simulink model "MIL_VehicleTestEnvironment_MG_DCT_19a"  (Simulink 9.3)
settings: Solver=ode4  StartTime=0.0  StopTime=20  FixedStep=0.001  MaxStep=0.005  RelTol=1e-3  EnableMultiTasking=on
model workspace (MAT data in the model file):
  CGFrntAxleDist = Simulink.Parameter
  CGFrntAxleDist.Value = 1.024
  CGFrntAxleDist.Description = ' the longitudinal distance from the center of gravity to front axle, [m]'
  CGFrntAxleDist.DataType = 'auto'
  CGFrntAxleDist.Dimensions = [1 1]
  CGHght = Simulink.Parameter
  CGHght.Value = 0.654
  CGHght.Description = 'the height of the center of gravity from ground, [m]'
  CGHght.DataType = 'auto'
  CGHght.Dimensions = [1 1]
  CGRearAxleDist = Simulink.Parameter
  CGRearAxleDist.Value = 1.536
  CGRearAxleDist.Description = 'the longitudinal distance from the center of gravity to rear axle, [m]'
  CGRearAxleDist.DataType = 'auto'
  CGRearAxleDist.Dimensions = [1 1]
  Clu1EffRad = Simulink.Parameter
  Clu1EffRad.Value = 0.1847
  Clu1EffRad.Description = 'the diameter of outer circle of clutch 1, [m]'
  Clu1EffRad.DataType = 'auto'
  Clu1EffRad.Dimensions = [1 1]
  Clu1FricCoefMap = Simulink.Parameter
  Clu1FricCoefMap.Value = [0  0.11; 100  0.1221; 300  0.1266; 1000  0.1348; 1700  0.1435]
  Clu1FricCoefMap.Description = 'the friction coefficent of clutch 1 as a function of angular velocity difference [rpm]'
  Clu1FricCoefMap.DataType = 'auto'
  Clu1FricCoefMap.Dimensions = [5 2]
  Clu1FricSurfNum = Simulink.Parameter
  Clu1FricSurfNum.Value = 6
  Clu1FricSurfNum.Description = 'the amount of friction surfaces on clutch 1'
  Clu1FricSurfNum.DataType = 'auto'
  Clu1FricSurfNum.Dimensions = [1 1]
  Clu1OutpInrt = Simulink.Parameter
  Clu1OutpInrt.Value = 0.003321
  Clu1OutpInrt.Description = 'inertia of Clutch output part 1, [kg*m*m]'
  Clu1OutpInrt.DataType = 'auto'
  Clu1OutpInrt.Dimensions = [1 1]
  Clu1PMin = Simulink.Parameter
  Clu1PMin.Value = 1.3
  Clu1PMin.DataType = 'auto'
  Clu1PMin.Dimensions = [1 1]
  Clu1PresArea = Simulink.Parameter
  Clu1PresArea.Value = 0.0035
  Clu1PresArea.Description = 'the effected area of the oil pressure on clutch 1, [m*m] '
  Clu1PresArea.DataType = 'auto'
  Clu1PresArea.Dimensions = [1 1]
  Clu1SprFor = Simulink.Parameter
  Clu1SprFor.Value = 809
  Clu1SprFor.Description = 'the seperate spring force of clutch 1, [N]'
  Clu1SprFor.DataType = 'auto'
  Clu1SprFor.Dimensions = [1 1]
  Clu1StatFricCoef = Simulink.Parameter
  Clu1StatFricCoef.Value = 0.12
  Clu1StatFricCoef.Description = 'the static friction peak coefficient of clutch 2, no less than the kinetic friction coefficient at 0 velocity'
  Clu1StatFricCoef.DataType = 'auto'
  Clu1StatFricCoef.Dimensions = [1 1]
  Clu2EffRad = Simulink.Parameter
  Clu2EffRad.Value = 0.1397
  Clu2EffRad.Description = 'the effected radius of clutch 2, [m]'
  Clu2EffRad.DataType = 'auto'
  Clu2EffRad.Dimensions = [1 1]
  Clu2FricCoefMap = Simulink.Parameter
  Clu2FricCoefMap.Value = [0  0.11; 100  0.1225; 300  0.1274; 1000  0.1348; 1700  0.1397]
  Clu2FricCoefMap.Description = 'the friction coefficent of clutch 2 as a function of angular velocity difference [rpm]'
  Clu2FricCoefMap.DataType = 'auto'
  Clu2FricCoefMap.Dimensions = [5 2]
  Clu2FricSurfNum = Simulink.Parameter
  Clu2FricSurfNum.Value = 8
  Clu2FricSurfNum.Description = 'the amount of friction surfaces on clutch 2'
  Clu2FricSurfNum.DataType = 'auto'
  Clu2FricSurfNum.Dimensions = [1 1]
  Clu2OutpInrt = Simulink.Parameter
  Clu2OutpInrt.Value = 0.002617
  Clu2OutpInrt.Description = 'inertia of Clutch output part 2, [kg*m*m]'
  Clu2OutpInrt.DataType = 'auto'
  Clu2OutpInrt.Dimensions = [1 1]
  Clu2PMin = Simulink.Parameter
  Clu2PMin.Value = 1.3
  Clu2PMin.DataType = 'auto'
  Clu2PMin.Dimensions = [1 1]
  Clu2PresArea = Simulink.Parameter
  Clu2PresArea.Value = 0.0035
  Clu2PresArea.Description = 'the effected area of the oil pressure on clutch 2, [m*m] '
  Clu2PresArea.DataType = 'auto'
  Clu2PresArea.Dimensions = [1 1]
  Clu2SprFor = Simulink.Parameter
  Clu2SprFor.Value = 809
  Clu2SprFor.Description = 'the seperate spring force of clutch 2, [N]'
  Clu2SprFor.DataType = 'auto'
  Clu2SprFor.Dimensions = [1 1]
  Clu2StatFricCoef = Simulink.Parameter
  Clu2StatFricCoef.Value = 0.12
  Clu2StatFricCoef.Description = 'the static friction peak coefficient of clutch 2, no less than the kinetic friction coefficient at 0 velocity'
  Clu2StatFricCoef.DataType = 'auto'
  Clu2StatFricCoef.Dimensions = [1 1]
  CluInpInrt = Simulink.Parameter
  CluInpInrt.Value = 0.0225
  CluInpInrt.Description = 'inertia of Clutch input part, [kg*m*m]'
  CluInpInrt.DataType = 'auto'
  CluInpInrt.Dimensions = [1 1]
  CluSoln1LineI = Simulink.Parameter
  CluSoln1LineI.Value = [200 400 600 800 950]
  CluSoln1LineI.Description = 'mA
    | '
  CluSoln1LineI.DataType = 'auto'
  CluSoln1LineI.Dimensions = [1 5]
  CluSoln1LineP = Simulink.Parameter
  CluSoln1LineP.Value = [0 2.5 8.85 15.77 20]
  CluSoln1LineP.Description = 'bar/1000'
  CluSoln1LineP.DataType = 'auto'
  CluSoln1LineP.Dimensions = [1 5]
  CluSoln2LineI = Simulink.Parameter
  CluSoln2LineI.Value = [200 400 600 800 950]
  CluSoln2LineI.Description = 'mA
    | '
  CluSoln2LineI.DataType = 'auto'
  CluSoln2LineI.Dimensions = [1 5]
  CluSoln2LineP = Simulink.Parameter
  CluSoln2LineP.Value = [0 2.5 8.85 15.77 20]
  CluSoln2LineP.Description = 'bar/1000'
  CluSoln2LineP.DataType = 'auto'
  CluSoln2LineP.Dimensions = [1 5]
  DiffDampCoef = Simulink.Parameter
  DiffDampCoef.Value = 0.001
  DiffDampCoef.Description = 'the inertia of final drive gear and differential, [kg*m*m]'
  DiffDampCoef.DataType = 'auto'
  DiffDampCoef.Dimensions = [1 1]
  DiffInrt = Simulink.Parameter
  DiffInrt.Value = 0.0448
  DiffInrt.Description = 'the inertia of final drive gear and differential, [kg*m*m]'
  DiffInrt.DataType = 'auto'
  DiffInrt.Dimensions = [1 1]
  EngDampCoef = Simulink.Parameter
  EngDampCoef.Value = 0.03
  EngDampCoef.Description = 'the damper coefficent of engine shaft, [N*m*s/rad]'
  EngDampCoef.DataType = 'auto'
  EngDampCoef.Dimensions = [1 1]
  EngFuelCnsPerKWhMapCns = Simulink.Parameter
  EngFuelCnsPerKWhMapCns.Value = [300 300 300 300 300 300 300 300 300 300 300 300 ... (5858 elements, 101x58)]
  EngFuelCnsPerKWhMapCns.DataType = 'auto'
  EngFuelCnsPerKWhMapCns.Dimensions = [101 58]
  EngFuelCnsPerKWhMapSpdIndx = Simulink.Parameter
  EngFuelCnsPerKWhMapSpdIndx.Value = [800 900 1000 1100 1200 1300 1400 1500 1600 1700 1800 1900 2000 2100 2200 2300 2400 2500 2600 2700 2800 2900 3000 3100 3200 3300 3400 3500 3600 3700 3800 3900 4000 4100 4200 4300 4400 4500 4600 4700 4800 4900 5000 5100 5200 5300 5400 5500 5600 5700 5800 5900 6000 6100 6200 6300 6400 6500]
  EngFuelCnsPerKWhMapSpdIndx.DataType = 'auto'
  EngFuelCnsPerKWhMapSpdIndx.Dimensions = [1 58]
  EngFuelCnsPerKWhMapThrtIndx = Simulink.Parameter
  EngFuelCnsPerKWhMapThrtIndx.Value = [0 1 2 3 4 5 6 7 8 9 10 11 12 13 14 15 16 17 18 19 20 21 22 23 24 25 26 27 28 29 30 31 32 33 34 35 36 37 38 39 40 41 42 43 44 45 46 47 48 49 50 51 52 53 54 55 56 57 58 59 60 61 62 63 64 65 66 67 68 69 70 71 72 73 74 75 76 77 78 79 80 81 82 83 84 85 86 87 88 89 90 91 92 93 94 95 96 97 98 99 100]
  EngFuelCnsPerKWhMapThrtIndx.DataType = 'auto'
  EngFuelCnsPerKWhMapThrtIndx.Dimensions = [1 101]
  EngFuelCnsPerSecMapCns = Simulink.Parameter
  EngFuelCnsPerSecMapCns.Value = [0.08 0.2 0.3 0.32 0.34 0.37 0.39 0.41 0.43 0.46 0.48 0.5 ... (494 elements, 26x19)]
  EngFuelCnsPerSecMapCns.DataType = 'auto'
  EngFuelCnsPerSecMapCns.Dimensions = [26 19]
  EngFuelCnsPerSecMapSpdIndx = Simulink.Parameter
  EngFuelCnsPerSecMapSpdIndx.Value = [600 800 1000 1200 1400 1600 1800 2000 2200 2400 2800 3200 3600 4000 4400 4800 5200 5600 5800]
  EngFuelCnsPerSecMapSpdIndx.DataType = 'auto'
  EngFuelCnsPerSecMapSpdIndx.Dimensions = [1 19]
  EngFuelCnsPerSecMapThrtIndx = Simulink.Parameter
  EngFuelCnsPerSecMapThrtIndx.Value = [0 4 8 12 16 20 24 28 32 36 40 44 48 52 56 60 64 68 72 76 80 84 88 92 96 100]
  EngFuelCnsPerSecMapThrtIndx.DataType = 'auto'
  EngFuelCnsPerSecMapThrtIndx.Dimensions = [1 26]
  EngFuelRateMapPwrIndx = Simulink.Parameter
  EngFuelRateMapPwrIndx.Value = [0 1 2 3 4 5 6 7 8 9 10 11 12 13 14 15 16 17 18 19 20 21 22 23 24 25 26 27 28 29 30 31 32 33 34 35 36 37 38 39 40 41 42 43 44 45 46 47 48 49 50 51 52 53 54 55 56 57 58 59 60 61 62 63 64 65 66 67 68 69 70 71 72 73 74 75 76 77 78 79 80 81 82 83 84 85 86 87 88 89 90 91 92 93 94 95 96 97 98 99 100 101 102 103 104 105 106 107 108 109 110 111 112 113 114 115 116 117 118 119 120 121 122 123 124 125 126 127 128 129 130 131 132 133 134 135 136 137 138 139 140 141 142 143 144 145 146 147 148 149 150 151 152 153 154 155 156 157 158 159 160 161]
  EngFuelRateMapPwrIndx.DataType = 'auto'
  EngFuelRateMapPwrIndx.Dimensions = [1 162]
  EngFuelRateMapRate = Simulink.Parameter
  EngFuelRateMapRate.Value = [299.999982085 300.000046004 299.999957683 299.999715746 300.001791195 299.994024584 300.011592336 299.999851192 299.918999195 299.430328902 286.286371749 262.121506938 ... (9396 elements, 162x58)]
  EngFuelRateMapRate.DataType = 'auto'
  EngFuelRateMapRate.Dimensions = [162 58]
  EngFuelRateMapSpdIndx = Simulink.Parameter
  EngFuelRateMapSpdIndx.Value = [800 900 1000 1100 1200 1300 1400 1500 1600 1700 1800 1900 2000 2100 2200 2300 2400 2500 2600 2700 2800 2900 3000 3100 3200 3300 3400 3500 3600 3700 3800 3900 4000 4100 4200 4300 4400 4500 4600 4700 4800 4900 5000 5100 5200 5300 5400 5500 5600 5700 5800 5900 6000 6100 6200 6300 6400 6500]
  EngFuelRateMapSpdIndx.DataType = 'auto'
  EngFuelRateMapSpdIndx.Dimensions = [1 58]
  EngIdleSpd = Simulink.Parameter
  EngIdleSpd.Value = 750
  EngIdleSpd.Description = 'the rated idle speed of engine, [rpm]'
  EngIdleSpd.DataType = 'auto'
  EngIdleSpd.Dimensions = [1 1]
  EngInrt = Simulink.Parameter
  EngInrt.Value = 0.2
  EngInrt.Description = 'the inertia of engine crank shaft and flywheel, [kg*m*m] '
  EngInrt.DataType = 'auto'
  EngInrt.Dimensions = [1 1]
  EngPwrMax = Simulink.Parameter
  EngPwrMax.Value = 162
  EngPwrMax.Description = ' maximum engine power, [kW]'
  EngPwrMax.DataType = 'auto'
  EngPwrMax.Dimensions = [1 1]
  EngSpdMax = Simulink.Parameter
  EngSpdMax.Value = 6500
  EngSpdMax.Description = 'maximum engine speed, [rpm]'
  EngSpdMax.DataType = 'auto'
  EngSpdMax.Dimensions = [1 1]
  EngTqExtChartc = Simulink.Parameter
  EngTqExtChartc.Value = [0 0 118.17 213.22 253 289.28 303.52 321 337.08 350 350 350 350 350 337.32 323.08 306.7 267.43 228.27 144 -80]
  EngTqExtChartc.DataType = 'auto'
  EngTqExtChartc.Dimensions = [1 21]
  EngTqMapSpdIndx = Simulink.Parameter
  EngTqMapSpdIndx.Value = [0 400 517 633 750 1107 1463 1820 2177 2533 2890 3247 3603 3960 4317 4673 5030 5387 5743 6100 6500]
  EngTqMapSpdIndx.Description = 'the speed index of engine universal characteristics, [rpm]'
  EngTqMapSpdIndx.DataType = 'auto'
  EngTqMapSpdIndx.Dimensions = [1 21]
  EngTqMapThrtIndx = Simulink.Parameter
  EngTqMapThrtIndx.Value = [0 10 20 30 40 50 60 70 80 90 100]
  EngTqMapThrtIndx.Description = 'the throttle index of engine universal characteristics, [%]'
  EngTqMapThrtIndx.DataType = 'auto'
  EngTqMapThrtIndx.Dimensions = [1 11]
  EngTqMapTq = Simulink.Parameter
  EngTqMapTq.Value = [0 0 0 0 0 0 0 0 0 0 0 0 ... (231 elements, 11x21)]
  EngTqMapTq.Description = 'torque map of engine universal characteristics, 11*20, [Nm]'
  EngTqMapTq.DataType = 'auto'
  EngTqMapTq.Dimensions = [11 21]
  EngTqMax = Simulink.Parameter
  EngTqMax.Value = 350
  EngTqMax.Description = 'maximum torque of engine, [Nm]'
  EngTqMax.DataType = 'auto'
  EngTqMax.Dimensions = [1 1]
  FinlGearRat1 = Simulink.Parameter
  FinlGearRat1.Value = 4.28
  FinlGearRat1.Description = 'the gear ratio of final drive 1'
  FinlGearRat1.DataType = 'auto'
  FinlGearRat1.Dimensions = [1 1]
  FinlGearRat2 = Simulink.Parameter
  FinlGearRat2.Value = 2.85
  FinlGearRat2.Description = 'the gear ratio of final drive 2'
  FinlGearRat2.DataType = 'auto'
  FinlGearRat2.Dimensions = [1 1]
  Fork13ActrAr = Simulink.Parameter
  Fork13ActrAr.Value = 400
  Fork13ActrAr.Description = 'mm^2'
  Fork13ActrAr.DataType = 'auto'
  Fork13ActrAr.Dimensions = [1 1]
  Fork1PosnA = Simulink.Parameter
  Fork1PosnA.Value = 795
  Fork1PosnA.DataType = 'uint16'
  Fork1PosnA.Dimensions = [1 1]
  Fork1PosnB = Simulink.Parameter
  Fork1PosnB.Value = 249
  Fork1PosnB.DataType = 'uint16'
  Fork1PosnB.Dimensions = [1 1]
  Fork1PosnNeut = Simulink.Parameter
  Fork1PosnNeut.Value = 513
  Fork1PosnNeut.DataType = 'uint16'
  Fork1PosnNeut.Dimensions = [1 1]
  Fork1PosnSyncA = Simulink.Parameter
  Fork1PosnSyncA.Value = 630
  Fork1PosnSyncA.DataType = 'uint16'
  Fork1PosnSyncA.Dimensions = [1 1]
  Fork1PosnSyncB = Simulink.Parameter
  Fork1PosnSyncB.Value = 410
  Fork1PosnSyncB.DataType = 'uint16'
  Fork1PosnSyncB.Dimensions = [1 1]
  Fork24ActrAr = Simulink.Parameter
  Fork24ActrAr.Value = 400
  Fork24ActrAr.DataType = 'auto'
  Fork24ActrAr.Dimensions = [1 1]
  Fork2PosnA = Simulink.Parameter
  Fork2PosnA.Value = 798
  Fork2PosnA.DataType = 'uint16'
  Fork2PosnA.Dimensions = [1 1]
  Fork2PosnB = Simulink.Parameter
  Fork2PosnB.Value = 228
  Fork2PosnB.DataType = 'uint16'
  Fork2PosnB.Dimensions = [1 1]
  Fork2PosnNeut = Simulink.Parameter
  Fork2PosnNeut.Value = 495
  Fork2PosnNeut.DataType = 'uint16'
  Fork2PosnNeut.Dimensions = [1 1]
  Fork2PosnSyncA = Simulink.Parameter
  Fork2PosnSyncA.Value = 610
  Fork2PosnSyncA.DataType = 'uint16'
  Fork2PosnSyncA.Dimensions = [1 1]
  Fork2PosnSyncB = Simulink.Parameter
  Fork2PosnSyncB.Value = 390
  Fork2PosnSyncB.DataType = 'uint16'
  Fork2PosnSyncB.Dimensions = [1 1]
  Fork3PosnA = Simulink.Parameter
  Fork3PosnA.Value = 820
  Fork3PosnA.DataType = 'uint16'
  Fork3PosnA.Dimensions = [1 1]
  Fork3PosnB = Simulink.Parameter
  Fork3PosnB.Value = 218
  Fork3PosnB.DataType = 'uint16'
  Fork3PosnB.Dimensions = [1 1]
  Fork3PosnNeut = Simulink.Parameter
  Fork3PosnNeut.Value = 515
  Fork3PosnNeut.DataType = 'uint16'
  Fork3PosnNeut.Dimensions = [1 1]
  Fork3PosnSyncA = Simulink.Parameter
  Fork3PosnSyncA.Value = 630
  Fork3PosnSyncA.DataType = 'uint16'
  Fork3PosnSyncA.Dimensions = [1 1]
  Fork3PosnSyncB = Simulink.Parameter
  Fork3PosnSyncB.Value = 410
  Fork3PosnSyncB.DataType = 'uint16'
  Fork3PosnSyncB.Dimensions = [1 1]
  Fork4PosnA = Simulink.Parameter
  Fork4PosnA.Value = 810
  Fork4PosnA.DataType = 'uint16'
  Fork4PosnA.Dimensions = [1 1]
  Fork4PosnB = Simulink.Parameter
  Fork4PosnB.Value = 224
  Fork4PosnB.DataType = 'uint16'
  Fork4PosnB.Dimensions = [1 1]
  Fork4PosnNeut = Simulink.Parameter
  Fork4PosnNeut.Value = 513
  Fork4PosnNeut.DataType = 'uint16'
  Fork4PosnNeut.Dimensions = [1 1]
  Fork4PosnSyncA = Simulink.Parameter
  Fork4PosnSyncA.Value = 630
  Fork4PosnSyncA.DataType = 'uint16'
  Fork4PosnSyncA.Dimensions = [1 1]
  Fork4PosnSyncB = Simulink.Parameter
  Fork4PosnSyncB.Value = 410
  Fork4PosnSyncB.DataType = 'uint16'
  Fork4PosnSyncB.Dimensions = [1 1]
  Fork6RActrAr = Simulink.Parameter
  Fork6RActrAr.Value = 400
  Fork6RActrAr.Description = 'mm^2'
  Fork6RActrAr.DataType = 'auto'
  Fork6RActrAr.Dimensions = [1 1]
  ForkMass = Simulink.Parameter
  ForkMass.Value = 0.5
  ForkMass.Description = 'the mass of fork and fork shaft'
  ForkMass.DataType = 'auto'
  ForkMass.Dimensions = [1 1]
  ForkN5ActrAr = Simulink.Parameter
  ForkN5ActrAr.Value = 400
  ForkN5ActrAr.Description = 'mm^2'
  ForkN5ActrAr.DataType = 'auto'
  ForkN5ActrAr.Dimensions = [1 1]
  GearRat = Simulink.Parameter
  GearRat.Value = [3.25 1.88 1.21 0.9 1.03 0.79 4.33]
  GearRat.Description = 'the gear ratio at gear 1-7&R'
  GearRat.DataType = 'auto'
  GearRat.Dimensions = [1 7]
  HalfShafInrt = Simulink.Parameter
  HalfShafInrt.Value = 0.0068
  HalfShafInrt.Description = 'inertia of two half shaft, [kg*m*m]'
  HalfShafInrt.DataType = 'auto'
  HalfShafInrt.Dimensions = [1 1]
  IdleGearInrt = Simulink.Parameter
  IdleGearInrt.Value = [0.00367 0.00297 0.0018 0.00123 0.00086 0.00056 0.0018]
  IdleGearInrt.Description = '% inertia of idle gear of gear 1-7&R, [kg*m*m]'
  IdleGearInrt.DataType = 'auto'
  IdleGearInrt.Dimensions = [1 7]
  InpShaf1DampCoef = Simulink.Parameter
  InpShaf1DampCoef.Value = 0.001
  InpShaf1DampCoef.DataType = 'auto'
  InpShaf1DampCoef.Dimensions = [1 1]
  InpShaf1Inrt = Simulink.Parameter
  InpShaf1Inrt.Value = 0.0046
  InpShaf1Inrt.Description = 'the inertia of input shaft 1, including the gears on the shaft, [kg*m*m]'
  InpShaf1Inrt.DataType = 'auto'
  InpShaf1Inrt.Dimensions = [1 1]
  InpShaf2DampCoef = Simulink.Parameter
  InpShaf2DampCoef.Value = 0.001
  InpShaf2DampCoef.DataType = 'auto'
  InpShaf2DampCoef.Dimensions = [1 1]
  InpShaf2Inrt = Simulink.Parameter
  InpShaf2Inrt.Value = 0.0033
  InpShaf2Inrt.Description = ' the inertia of input shaft 2, including the gears on the shaft, [kg*m*m]'
  InpShaf2Inrt.DataType = 'auto'
  InpShaf2Inrt.Dimensions = [1 1]
  OutpShaf1DampCoef = Simulink.Parameter
  OutpShaf1DampCoef.Value = 0.001
  OutpShaf1DampCoef.DataType = 'auto'
  OutpShaf1DampCoef.Dimensions = [1 1]
  OutpShaf1Inrt = Simulink.Parameter
  OutpShaf1Inrt.Value = 0.0062
  OutpShaf1Inrt.Description = 'the inertia of output shaft 1, [kg*m*m]'
  OutpShaf1Inrt.DataType = 'auto'
  OutpShaf1Inrt.Dimensions = [1 1]
  OutpShaf2DampCoef = Simulink.Parameter
  OutpShaf2DampCoef.Value = 0.001
  OutpShaf2DampCoef.DataType = 'auto'
  OutpShaf2DampCoef.Dimensions = [1 1]
  OutpShaf2Inrt = Simulink.Parameter
  OutpShaf2Inrt.Value = 0.0085
  OutpShaf2Inrt.Description = 'the inertia of output shaft 2, [kg*m*m]'
  OutpShaf2Inrt.DataType = 'auto'
  OutpShaf2Inrt.Dimensions = [1 1]
  RoadSlop = Simulink.Parameter
  RoadSlop.Value = 0
  RoadSlop.Description = 'road slop gradient, [deg]'
  RoadSlop.DataType = 'auto'
  RoadSlop.Dimensions = [1 1]
  ShiftSoln1LineI = Simulink.Parameter
  ShiftSoln1LineI.Value = [0 1000 2000]
  ShiftSoln1LineI.Description = 'mA
    | '
  ShiftSoln1LineI.DataType = 'auto'
  ShiftSoln1LineI.Dimensions = [1 3]
  ShiftSoln1LineP = Simulink.Parameter
  ShiftSoln1LineP.Value = [0 10 20]
  ShiftSoln1LineP.Description = 'bar/1000'
  ShiftSoln1LineP.DataType = 'auto'
  ShiftSoln1LineP.Dimensions = [1 3]
  ShiftSoln2LineI = Simulink.Parameter
  ShiftSoln2LineI.Value = [0 1000 2000]
  ShiftSoln2LineI.Description = 'mA
    | '
  ShiftSoln2LineI.DataType = 'auto'
  ShiftSoln2LineI.Dimensions = [1 3]
  ShiftSoln2LineP = Simulink.Parameter
  ShiftSoln2LineP.Value = [0 10 20]
  ShiftSoln2LineP.Description = 'bar/1000'
  ShiftSoln2LineP.DataType = 'auto'
  ShiftSoln2LineP.Dimensions = [1 3]
  SynrConeAngl = Simulink.Parameter
  SynrConeAngl.Value = 5
  SynrConeAngl.Description = 'the cone angle of a synchronizer, [rad]
    | 7.5'
  SynrConeAngl.DataType = 'auto'
  SynrConeAngl.Dimensions = [1 1]
  SynrDetnForMax = Simulink.Parameter
  SynrDetnForMax.Value = 70
  SynrDetnForMax.Description = 'peak force of synchronizer''s detent, [N]'
  SynrDetnForMax.DataType = 'auto'
  SynrDetnForMax.Dimensions = [1 1]
  SynrDiaBig = Simulink.Parameter
  SynrDiaBig.Value = 0.0728
  SynrDiaBig.Description = 'the maximum diameter of synchronizer contact surface, [m]'
  SynrDiaBig.DataType = 'auto'
  SynrDiaBig.Dimensions = [1 1]
  SynrDiaSmal = Simulink.Parameter
  SynrDiaSmal.Value = 0.0676
  SynrDiaSmal.Description = 'the minimum diameter of synchronizer contact surface, [m]'
  SynrDiaSmal.DataType = 'auto'
  SynrDiaSmal.Dimensions = [1 1]
  SynrDplDog = Simulink.Parameter
  SynrDplDog.Value = 10.514
  SynrDplDog.DataType = 'auto'
  SynrDplDog.Dimensions = [1 1]
  SynrDplEngd = Simulink.Parameter
  SynrDplEngd.Value = 13.514
  SynrDplEngd.DataType = 'auto'
  SynrDplEngd.Dimensions = [1 1]
  SynrDplFinshd = Simulink.Parameter
  SynrDplFinshd.Value = 18.211
  SynrDplFinshd.DataType = 'auto'
  SynrDplFinshd.Dimensions = [1 1]
  SynrDplSync = Simulink.Parameter
  SynrDplSync.Value = 5.074
  SynrDplSync.DataType = 'auto'
  SynrDplSync.Dimensions = [1 1]
  SynrFricCoef = Simulink.Parameter
  SynrFricCoef.Value = [0  0.35; 1000000  0.35]
  SynrFricCoef.Description = 'the friction coefficient of synchronizer contact surface'
  SynrFricCoef.DataType = 'auto'
  SynrFricCoef.Dimensions = [2 2]
  SynrNotchWidth = Simulink.Parameter
  SynrNotchWidth.Value = 18
  SynrNotchWidth.DataType = 'auto'
  SynrNotchWidth.Dimensions = [1 1]
  SynrVcosFricCoeff = Simulink.Parameter
  SynrVcosFricCoeff.Value = 300
  SynrVcosFricCoeff.DataType = 'auto'
  SynrVcosFricCoeff.Dimensions = [1 1]
  TireForMax = Simulink.Parameter
  TireForMax.Value = 16000
  TireForMax.Description = 'maximum tire longitudinal force, [N]'
  TireForMax.DataType = 'auto'
  TireForMax.Dimensions = [1 1]
  TireLoadRatd = Simulink.Parameter
  TireLoadRatd.Value = 20000
  TireLoadRatd.Description = 'rated tire vertical load, [N]'
  TireLoadRatd.DataType = 'auto'
  TireLoadRatd.Dimensions = [1 1]
  TireRad = Simulink.Parameter
  TireRad.Value = 0.346
  TireRad.Description = 'tire radius, [m]'
  TireRad.DataType = 'auto'
  TireRad.Dimensions = [1 1]
  TireRelxLen = Simulink.Parameter
  TireRelxLen.Value = 0.2
  TireRelxLen.Description = 'tire relaxation length at rated load, [m]'
  TireRelxLen.DataType = 'auto'
  TireRelxLen.Dimensions = [1 1]
  TireRollRest = Simulink.Parameter
  TireRollRest.Value = 0.015
  TireRollRest.Description = 'rolling resistance coefficient'
  TireRollRest.DataType = 'auto'
  TireRollRest.Dimensions = [1 1]
  TireSlipPeak = Simulink.Parameter
  TireSlipPeak.Value = 10
  TireSlipPeak.Description = 'slip at peak force at rated load, [%]'
  TireSlipPeak.DataType = 'auto'
  TireSlipPeak.Dimensions = [1 1]
  VBS1R = Simulink.Parameter
  VBS1R.Value = 4.15
  VBS1R.Description = 'Ohm'
  VBS1R.DataType = 'auto'
  VBS1R.Dimensions = [1 1]
  VBS2R = Simulink.Parameter
  VBS2R.Value = 4.15
  VBS2R.Description = 'Ohm'
  VBS2R.DataType = 'auto'
  VBS2R.Dimensions = [1 1]
  VBS3R = Simulink.Parameter
  VBS3R.Value = 4.17
  VBS3R.Description = 'Ohm'
  VBS3R.DataType = 'auto'
  VBS3R.Dimensions = [1 1]
  VBS4R = Simulink.Parameter
  VBS4R.Value = 4.17
  VBS4R.Description = 'Ohm'
  VBS4R.DataType = 'auto'
  VBS4R.Dimensions = [1 1]
  VFS1R = Simulink.Parameter
  VFS1R.Value = 5.2
  VFS1R.Description = 'Ohm'
  VFS1R.DataType = 'auto'
  VFS1R.Dimensions = [1 1]
  VFS2R = Simulink.Parameter
  VFS2R.Value = 5.2
  VFS2R.Description = 'Ohm'
  VFS2R.DataType = 'auto'
  VFS2R.Dimensions = [1 1]
  VehAirDragCoef = Simulink.Parameter
  VehAirDragCoef.Value = 0.4
  VehAirDragCoef.Description = 'the vehicle''s air drag coefficient, [-]'
  VehAirDragCoef.DataType = 'auto'
  VehAirDragCoef.Dimensions = [1 1]
  VehDecMax = Simulink.Parameter
  VehDecMax.Value = 20
  VehDecMax.Description = 'maximum vehicle deceleration with 100% brake pedal tapped, [m/s/s]'
  VehDecMax.DataType = 'auto'
  VehDecMax.Dimensions = [1 1]
  VehFrntArea = Simulink.Parameter
  VehFrntArea.Value = 2.424
  VehFrntArea.Description = 'the vehicle''s frontal area, [m*m]'
  VehFrntArea.DataType = 'auto'
  VehFrntArea.Dimensions = [1 1]
  VehMass = Simulink.Parameter
  VehMass.Value = 1617
  VehMass.Description = 'vehicle mass, [kg]'
  VehMass.DataType = 'auto'
  VehMass.Dimensions = [1 1]
  VehSpdInit = Simulink.Parameter
  VehSpdInit.Value = 0
  VehSpdInit.Description = 'the initial vehicle speed at the beginning of simulation, [m/s]'
  VehSpdInit.DataType = 'auto'
  VehSpdInit.Dimensions = [1 1]
  WhlInrt = Simulink.Parameter
  WhlInrt.Value = 1.5
  WhlInrt.Description = 'inertia of a single wheel, [kg*m*m]'
  WhlInrt.DataType = 'auto'
  WhlInrt.Dimensions = [1 1]
undefined symbols (not defined in the file or in its folder): Clu1FricCoefMap, Clu2FricCoefMap, CluSoln1LineI, CluSoln1LineP, CluSoln2LineI, CluSoln2LineP, DiffDampCoef, EngFuelCnsPerSecMapCns, EngFuelCnsPerSecMapSpdIndx, EngFuelCnsPerSecMapThrtIndx, EngIdleSpd, EngSpdMax, EngTqExtChartc, EngTqMapSpdIndx, EngTqMapThrtIndx, EngTqMapTq, EngTqMax, Fork13ActrAr, Fork1PosnA, Fork1PosnB, Fork1PosnNeut, Fork1PosnSyncA, Fork1PosnSyncB, Fork24ActrAr, Fork2PosnA, Fork2PosnB, Fork2PosnNeut, Fork2PosnSyncA, Fork2PosnSyncB, Fork3PosnA, Fork3PosnB, Fork3PosnNeut, Fork3PosnSyncA, Fork3PosnSyncB, Fork4PosnA, Fork4PosnB, Fork4PosnNeut, Fork4PosnSyncA, Fork4PosnSyncB, Fork6RActrAr, ForkN5ActrAr, GearRat, HalfShafInrt, IdleGearInrt, InpShaf1DampCoef, InpShaf2DampCoef, OutpShaf1DampCoef, OutpShaf2DampCoef, ShiftSoln1LineI, ShiftSoln1LineP, ShiftSoln2LineI, ShiftSoln2LineP, SynrDiaBig, SynrDplDog, SynrDplEngd, SynrDplFinshd, SynrDplSync, SynrFricCoef, VBS1R, VBS2R ... (+6)
libraries: fl_lib x71, nesl_utility x34, sdl_lib x20, fl_ps_legacy_lib x8, simulink x5
(part 1 of 2)
settings Model: Creator=SHAW  LastModifiedBy=DELL
settings DataIOCC: LimitDataPoints=on  SignalLoggingSaveFormat=Dataset
settings DebuggingCC: UnderspecifiedInitializationDetection=Simplified  MergeDetectMultiDrivingBlocksExec=error  SolverPrmCheckMsg=warning  FcnCallInpInsideContextMsg=error
settings HardwareCC: ProdBitPerInt=16  ProdBitPerPointer=16  ProdBitPerSizeT=16  ProdBitPerPtrDiffT=16  ProdEndianess=BigEndian  ProdWordSize=16  ProdHWDeviceType=Freescale->S12x
settings GRTTargetCC: CombineOutputUpdateFcns=on  GRTInterface=off
settings ConfigComp: CovSFcnEnable=off
settings SimscapeCC: SimscapeNormalizeSystem=off

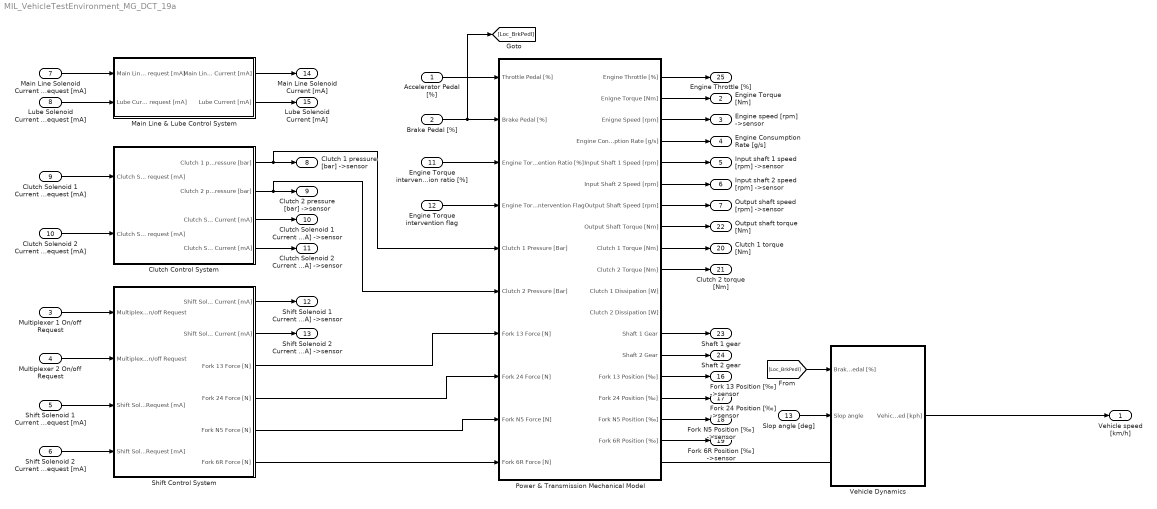
== system MIL_VehicleTestEnvironment_MG_DCT_19a ==
  Accelerator Pedal [%] : Inport
  Brake Pedal [%] : Inport  Port=2
  Multiplexer 1 On/off Request : Inport  Port=3
  Multiplexer 2 On/off Request : Inport  Port=4
  Shift Solenoid 1 Current Request [mA] : Inport  Port=5
  Shift Solenoid 2 Current Request [mA] : Inport  Port=6
  Main Line Solenoid Current request [mA] : Inport  Port=7
  Lube Solenoid Current request [mA] : Inport  Port=8
  Clutch Solenoid 1 Current request [mA] : Inport  Port=9
  Clutch Solenoid 2 Current request [mA] : Inport  Port=10
  Engine Torque intervention ratio [%] : Inport  Port=11
  Engine Torque intervention flag : Inport  Port=12
  Slop angle [deg] : Inport  Port=13
  Clutch Control System : Subsystem
  Main Line & Lube Control System : Subsystem
  "Power & Transmission Mechanical Model " : Subsystem
  Shift Control System : Subsystem
  Vehicle Dynamics : Subsystem
  Vehicle speed [km/h] : Outport  VectorParamsAs1DForOutWhenUnconnected=off
  Engine Torque [Nm] : Outport  Port=2  VectorParamsAs1DForOutWhenUnconnected=off
  Engine speed [rpm] ->sensor : Outport  Port=3  VectorParamsAs1DForOutWhenUnconnected=off
  Engine Consumption Rate [g/s] : Outport  Port=4  VectorParamsAs1DForOutWhenUnconnected=off
  Input shaft 1 speed [rpm] ->sensor : Outport  Port=5  VectorParamsAs1DForOutWhenUnconnected=off
  "Input shaft 2 speed [rpm] ->sensor " : Outport  Port=6  VectorParamsAs1DForOutWhenUnconnected=off
  Output shaft speed [rpm] ->sensor : Outport  Port=7  VectorParamsAs1DForOutWhenUnconnected=off
  Clutch 1 pressure [bar] ->sensor : Outport  Port=8  VectorParamsAs1DForOutWhenUnconnected=off
  Clutch 2 pressure [bar] ->sensor : Outport  Port=9  VectorParamsAs1DForOutWhenUnconnected=off
  Clutch Solenoid 1 Current [mA] ->sensor : Outport  Port=10  VectorParamsAs1DForOutWhenUnconnected=off
  Clutch Solenoid 2 Current [mA] ->sensor : Outport  Port=11  VectorParamsAs1DForOutWhenUnconnected=off
  Shift Solenoid 1 Current [mA] ->sensor : Outport  Port=12  VectorParamsAs1DForOutWhenUnconnected=off
  Shift Solenoid 2 Current [mA] ->sensor : Outport  Port=13  VectorParamsAs1DForOutWhenUnconnected=off
  Main Line Solenoid Current [mA] : Outport  Port=14  VectorParamsAs1DForOutWhenUnconnected=off
  Lube Solenoid Current [mA] : Outport  Port=15  VectorParamsAs1DForOutWhenUnconnected=off
  Fork 13 Position [‰] ->sensor : Outport  Port=16  VectorParamsAs1DForOutWhenUnconnected=off
  Fork 24 Position [‰] ->sensor : Outport  Port=17  VectorParamsAs1DForOutWhenUnconnected=off
  Fork N5 Position [‰] ->sensor : Outport  Port=18  VectorParamsAs1DForOutWhenUnconnected=off
  Fork 6R Position [‰] ->sensor : Outport  Port=19  VectorParamsAs1DForOutWhenUnconnected=off
  Clutch 1 torque [Nm] : Outport  Port=20  VectorParamsAs1DForOutWhenUnconnected=off
  Clutch 2 torque [Nm] : Outport  Port=21  VectorParamsAs1DForOutWhenUnconnected=off
  Output shaft torque [Nm] : Outport  Port=22  VectorParamsAs1DForOutWhenUnconnected=off
  Shaft 1 gear : Outport  Port=23  VectorParamsAs1DForOutWhenUnconnected=off
  Shaft 2 gear : Outport  Port=24  VectorParamsAs1DForOutWhenUnconnected=off
  Engine Throttle [%] : Outport  Port=25  VectorParamsAs1DForOutWhenUnconnected=off
  wires:
  Accelerator Pedal [%]/1 -> "Power & Transmission Mechanical Model "/1(Throttle Pedal [%])
  Brake Pedal [%]/1 -> [Loc_BrkPedl], "Power & Transmission Mechanical Model "/2(Brake Pedal [%])
  Engine Torque intervention ratio [%]/1 -> "Power & Transmission Mechanical Model "/3(Engine Torque Intervention Ratio [%])
  Engine Torque intervention flag/1 -> "Power & Transmission Mechanical Model "/4(Engine Torque Intervention Flag)
  "Power & Transmission Mechanical Model "/2(Enigne Torque [Nm]) -> Engine Torque [Nm]/1
  "Power & Transmission Mechanical Model "/3(Enigne Speed [rpm]) -> Engine speed [rpm] ->sensor/1
  "Power & Transmission Mechanical Model "/5(Input Shaft 1 Speed [rpm]) -> Input shaft 1 speed [rpm] ->sensor/1
  "Power & Transmission Mechanical Model "/6(Input Shaft 2 Speed [rpm]) -> "Input shaft 2 speed [rpm] ->sensor "/1
  "Power & Transmission Mechanical Model "/7(Output Shaft Speed [rpm]) -> Output shaft speed [rpm] ->sensor/1
  "Power & Transmission Mechanical Model "/9(Clutch 1 Torque [Nm]) -> Clutch 1 torque [Nm]/1
  "Power & Transmission Mechanical Model "/10(Clutch 2 Torque [Nm]) -> Clutch 2 torque [Nm]/1
  "Power & Transmission Mechanical Model "/13(Shaft 1 Gear) -> Shaft 1 gear/1
  "Power & Transmission Mechanical Model "/14(Shaft 2 Gear) -> Shaft 2 gear/1
  Vehicle Dynamics/1(Vehicle Speed [kph]) -> Vehicle speed [km/h]/1
  [Loc_BrkPedl] -> Vehicle Dynamics/1(Brake Pedal [%])
  "Power & Transmission Mechanical Model "/8(Output Shaft Torque [Nm]) -> Output shaft torque [Nm]/1
  Clutch Solenoid 2 Current request [mA]/1 -> Clutch Control System/2(Clutch Solenoid 2 Current request [mA])
  Clutch Solenoid 1 Current request [mA]/1 -> Clutch Control System/1(Clutch Solenoid 1 Current request [mA])
  Clutch Control System/3(Clutch Solenoid 1 Current [mA]) -> Clutch Solenoid 1 Current [mA] ->sensor/1
  Clutch Control System/4(Clutch Solenoid 2 Current [mA]) -> Clutch Solenoid 2 Current [mA] ->sensor/1
  Clutch Control System/1(Clutch 1 pressure [bar]) -> Clutch 1 pressure [bar] ->sensor/1, "Power & Transmission Mechanical Model "/5(Clutch 1 Pressure [Bar])
  Clutch Control System/2(Clutch 2 pressure [bar]) -> "Power & Transmission Mechanical Model "/6(Clutch 2 Pressure [Bar]), Clutch 2 pressure [bar] ->sensor/1
  Multiplexer 1 On/off Request/1 -> Shift Control System/1(Multiplexer 1 On/off Request)
  Shift Solenoid 1 Current Request [mA]/1 -> Shift Control System/3(Shift Solenoid 1 Current Request [mA])
  Shift Control System/1(Shift Solenoid 1 Current [mA]) -> Shift Solenoid 1 Current [mA] ->sensor/1
  Shift Control System/2(Shift Solenoid 2 Current [mA]) -> Shift Solenoid 2 Current [mA] ->sensor/1
  Shift Control System/6(Fork 6R Force [N]) -> "Power & Transmission Mechanical Model "/10(Fork 6R Force [N])
  Shift Control System/5(Fork N5 Force [N]) -> "Power & Transmission Mechanical Model "/9(Fork N5 Force [N])
  Shift Control System/4(Fork 24 Force [N]) -> "Power & Transmission Mechanical Model "/8(Fork 24 Force [N])
  Shift Control System/3(Fork 13 Force [N]) -> "Power & Transmission Mechanical Model "/7(Fork 13 Force [N])
  "Power & Transmission Mechanical Model "/15(Fork 13 Position [‰]) -> Fork 13 Position [‰] ->sensor/1
  "Power & Transmission Mechanical Model "/17(Fork N5 Position [‰]) -> Fork N5 Position [‰] ->sensor/1
  "Power & Transmission Mechanical Model "/16(Fork 24 Position [‰]) -> Fork 24 Position [‰] ->sensor/1
  "Power & Transmission Mechanical Model "/18(Fork 6R Position [‰]) -> Fork 6R Position [‰] ->sensor/1
  Slop angle [deg]/1 -> Vehicle Dynamics/2(Slop angle)
  Shift Solenoid 2 Current Request [mA]/1 -> Shift Control System/4(Shift Solenoid 2 Current Request [mA])
  Multiplexer 2 On/off Request/1 -> Shift Control System/2(Multiplexer 2 On/off Request)
  Main Line Solenoid Current request [mA]/1 -> Main Line & Lube Control System/1(Main Line Current request [mA])
  Lube Solenoid Current request [mA]/1 -> Main Line & Lube Control System/2(Lube Current request [mA])
  Main Line & Lube Control System/1(Main Line Current [mA]) -> Main Line Solenoid Current [mA]/1
  Main Line & Lube Control System/2(Lube Current [mA]) -> Lube Solenoid Current [mA]/1
  "Power & Transmission Mechanical Model "/1(Engine Throttle [%]) -> Engine Throttle [%]/1
  "Power & Transmission Mechanical Model "/4(Engine Consumption Rate [g/s]) -> Engine Consumption Rate [g/s]/1
  connections:
  Vehicle Dynamics/LConn1 -- "Power & Transmission Mechanical Model "/RConn1

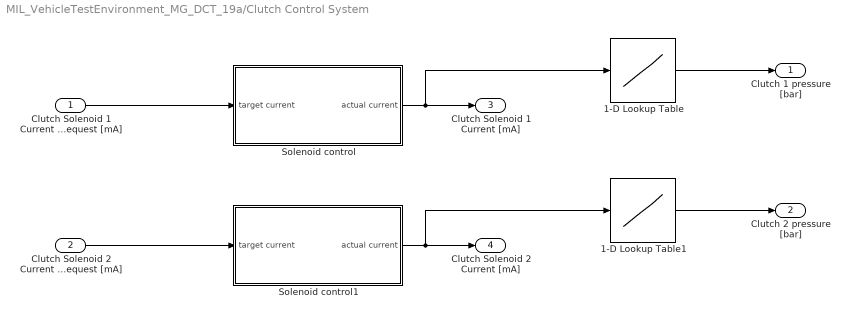
== system MIL_VehicleTestEnvironment_MG_DCT_19a/Clutch Control System ==
  Clutch Solenoid 1 Current request [mA] : Inport
  Clutch Solenoid 2 Current request [mA] : Inport  Port=2
  1-D Lookup Table : Lookup_n-D  NumberOfTableDimensions=1  BreakpointsForDimension1=CluSoln1LineI  Table=CluSoln1LineP  ExtrapMethod=Clip  InternalRulePriority=Speed  RndMeth=Simplest  InputSameDT=on
  1-D Lookup Table1 : Lookup_n-D  NumberOfTableDimensions=1  BreakpointsForDimension1=CluSoln2LineI  Table=CluSoln2LineP  ExtrapMethod=Clip  InternalRulePriority=Speed  RndMeth=Simplest  InputSameDT=on
  Solenoid control : Subsystem
  Solenoid control1 : Subsystem
  Clutch 1 pressure [bar] : Outport  VectorParamsAs1DForOutWhenUnconnected=off
  Clutch 2 pressure [bar] : Outport  Port=2  VectorParamsAs1DForOutWhenUnconnected=off
  Clutch Solenoid 1 Current [mA] : Outport  Port=3  VectorParamsAs1DForOutWhenUnconnected=off
  Clutch Solenoid 2 Current [mA] : Outport  Port=4  VectorParamsAs1DForOutWhenUnconnected=off
  wires:
  Clutch Solenoid 1 Current request [mA]/1 -> Solenoid control/1(target current)
  Solenoid control/1(actual current) -> 1-D Lookup Table/1, Clutch Solenoid 1 Current [mA]/1
  1-D Lookup Table/1 -> Clutch 1 pressure [bar]/1
  Clutch Solenoid 2 Current request [mA]/1 -> Solenoid control1/1(target current)
  Solenoid control1/1(actual current) -> 1-D Lookup Table1/1, Clutch Solenoid 2 Current [mA]/1
  1-D Lookup Table1/1 -> Clutch 2 pressure [bar]/1

== system MIL_VehicleTestEnvironment_MG_DCT_19a/Main Line & Lube Control System ==
  Main Line Current request [mA] : Inport
  Lube Current request [mA] : Inport  Port=2
  Solenoid control : Subsystem
  Solenoid control1 : Subsystem
  Main Line Current [mA] : Outport  VectorParamsAs1DForOutWhenUnconnected=off
  Lube Current [mA] : Outport  Port=2  VectorParamsAs1DForOutWhenUnconnected=off
  wires:
  Solenoid control1/1(actual current) -> Lube Current [mA]/1
  Lube Current request [mA]/1 -> Solenoid control1/1(target current)
  Solenoid control/1(actual current) -> Main Line Current [mA]/1
  Main Line Current request [mA]/1 -> Solenoid control/1(target current)

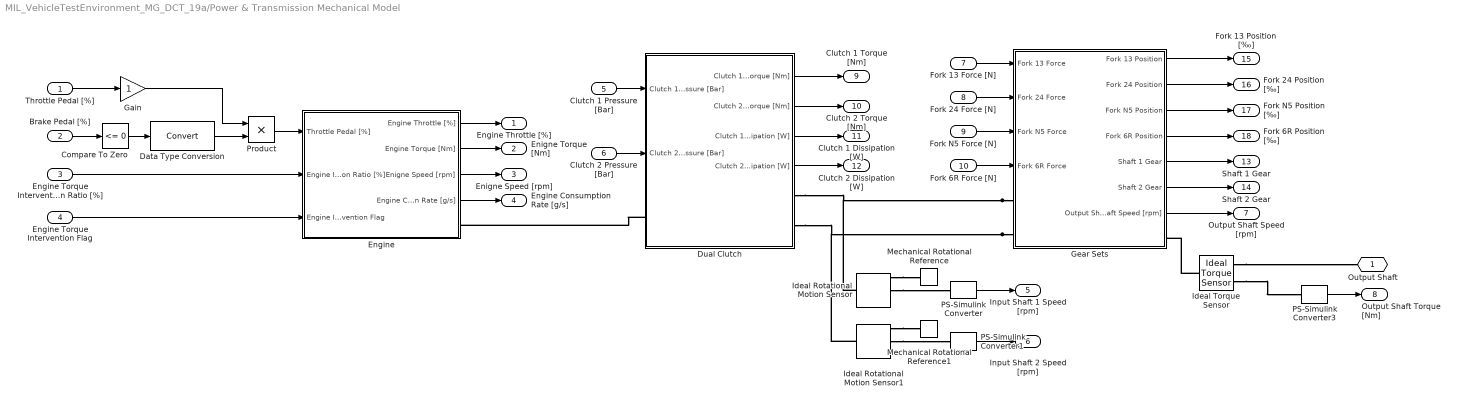
== system MIL_VehicleTestEnvironment_MG_DCT_19a/Power & Transmission Mechanical Model  ==
  Throttle Pedal [%] : Inport
  Brake Pedal [%] : Inport  Port=2
  Engine Torque Intervention Ratio [%] : Inport  Port=3
  Engine Torque Intervention Flag : Inport  Port=4
  Clutch 1 Pressure [Bar] : Inport  Port=5
  Clutch 2 Pressure [Bar] : Inport  Port=6
  Fork 13 Force [N] : Inport  Port=7
  Fork 24 Force [N] : Inport  Port=8
  Fork N5 Force [N] : Inport  Port=9
  Fork 6R Force [N] : Inport  Port=10
  Compare To Zero : simulink/Logic and Bit Operations/Compare To Zero  relop=<=  OutDataTypeStr=boolean
  Data Type Conversion : DataTypeConversion
  Dual Clutch : Subsystem
  Engine : Subsystem
  Gain : Gain
  Gear Sets : Subsystem
  Ideal Rotational Motion Sensor : fl_lib/Mechanical/Mechanical Sensors/Ideal Rotational Motion Sensor  wrap_angle=simscape.enum.onoff.off  offset=0 rad
  Ideal Rotational Motion Sensor1 : fl_lib/Mechanical/Mechanical Sensors/Ideal Rotational Motion Sensor  wrap_angle=simscape.enum.onoff.off  offset=0 rad
  Ideal Torque Sensor : fl_lib/Mechanical/Mechanical Sensors/Ideal Torque Sensor
  Mechanical Rotational Reference : fl_lib/Mechanical/Rotational Elements/Mechanical Rotational Reference
  Mechanical Rotational Reference1 : fl_lib/Mechanical/Rotational Elements/Mechanical Rotational Reference
  PS-Simulink Converter : nesl_utility/PS-Simulink Converter  PhysicalDomain=network_engine_domain  SubClassName=ps_output  LeftPortType=input  RightPortType=output  PseudoPeriodic=off  Frequencies=[]  Unit=rpm  AffineConversion=off
  PS-Simulink Converter1 : nesl_utility/PS-Simulink Converter  PhysicalDomain=network_engine_domain  SubClassName=ps_output  LeftPortType=input  RightPortType=output  PseudoPeriodic=off  Frequencies=[]  Unit=rpm  AffineConversion=off
  PS-Simulink Converter3 : nesl_utility/PS-Simulink Converter  PhysicalDomain=network_engine_domain  SubClassName=ps_output  LeftPortType=input  RightPortType=output  PseudoPeriodic=off  Frequencies=[]  Unit=N*m  AffineConversion=off
  Product : Product
  Output Shaft : PMIOPort  Side=Right
  Engine Throttle [%] : Outport  VectorParamsAs1DForOutWhenUnconnected=off
  Enigne Torque [Nm] : Outport  Port=2  VectorParamsAs1DForOutWhenUnconnected=off
  Enigne Speed [rpm] : Outport  Port=3  VectorParamsAs1DForOutWhenUnconnected=off
  Engine Consumption Rate [g/s] : Outport  Port=4  VectorParamsAs1DForOutWhenUnconnected=off
  Input Shaft 1 Speed [rpm] : Outport  Port=5  VectorParamsAs1DForOutWhenUnconnected=off
  Input Shaft 2 Speed [rpm] : Outport  Port=6  VectorParamsAs1DForOutWhenUnconnected=off
  Output Shaft Speed [rpm] : Outport  Port=7  VectorParamsAs1DForOutWhenUnconnected=off
  Output Shaft Torque [Nm] : Outport  Port=8  VectorParamsAs1DForOutWhenUnconnected=off
  Clutch 1 Torque [Nm] : Outport  Port=9  VectorParamsAs1DForOutWhenUnconnected=off
  Clutch 2 Torque [Nm] : Outport  Port=10  VectorParamsAs1DForOutWhenUnconnected=off
  Clutch 1 Dissipation [W] : Outport  Port=11  VectorParamsAs1DForOutWhenUnconnected=off
  Clutch 2 Dissipation [W] : Outport  Port=12  VectorParamsAs1DForOutWhenUnconnected=off
  Shaft 1 Gear : Outport  Port=13  VectorParamsAs1DForOutWhenUnconnected=off
  Shaft 2 Gear : Outport  Port=14  VectorParamsAs1DForOutWhenUnconnected=off
  Fork 13 Position [‰] : Outport  Port=15  VectorParamsAs1DForOutWhenUnconnected=off
  Fork 24 Position [‰] : Outport  Port=16  VectorParamsAs1DForOutWhenUnconnected=off
  Fork N5 Position [‰] : Outport  Port=17  VectorParamsAs1DForOutWhenUnconnected=off
  Fork 6R Position [‰] : Outport  Port=18  VectorParamsAs1DForOutWhenUnconnected=off
  wires:
  Brake Pedal [%]/1 -> Compare To Zero/1
  Throttle Pedal [%]/1 -> Gain/1
  Compare To Zero/1 -> Data Type Conversion/1
  Product/1 -> Engine/1(Throttle Pedal [%])
  Engine Torque Intervention Ratio [%]/1 -> Engine/2(Engine Intervention Ratio [%])
  Engine Torque Intervention Flag/1 -> Engine/3(Engine Intervention Flag)
  Clutch 1 Pressure [Bar]/1 -> Dual Clutch/1(Clutch 1 Pressure [Bar])
  Clutch 2 Pressure [Bar]/1 -> Dual Clutch/2(Clutch 2 Pressure [Bar])
  Engine/2(Engine Torque [Nm]) -> Enigne Torque [Nm]/1
  Engine/3(Enigne Speed [rpm]) -> Enigne Speed [rpm]/1
  Dual Clutch/3(Clutch 1 Dissipation [W]) -> Clutch 1 Dissipation [W]/1
  Dual Clutch/2(Clutch 2 Torque [Nm]) -> Clutch 2 Torque [Nm]/1
  Dual Clutch/4(Clutch 2 Dissipation [W]) -> Clutch 2 Dissipation [W]/1
  Dual Clutch/1(Clutch 1 Torque [Nm]) -> Clutch 1 Torque [Nm]/1
  Gear Sets/5(Shaft 1 Gear) -> Shaft 1 Gear/1
  Gear Sets/6(Shaft 2 Gear) -> Shaft 2 Gear/1
  PS-Simulink Converter/1 -> Input Shaft 1 Speed [rpm]/1
  PS-Simulink Converter1/1 -> Input Shaft 2 Speed [rpm]/1
  Gear Sets/7(Output Shaft Speed [rpm]) -> Output Shaft Speed [rpm]/1
  PS-Simulink Converter3/1 -> Output Shaft Torque [Nm]/1
  Fork 13 Force [N]/1 -> Gear Sets/1(Fork 13 Force)
  Fork 24 Force [N]/1 -> Gear Sets/2(Fork 24 Force)
  Fork N5 Force [N]/1 -> Gear Sets/3(Fork N5 Force)
  Fork 6R Force [N]/1 -> Gear Sets/4(Fork 6R Force)
  Gain/1 -> Product/1
  Gear Sets/2(Fork 24 Position) -> Fork 24 Position [‰]/1
  Gear Sets/1(Fork 13 Position) -> Fork 13 Position [‰]/1
  Gear Sets/4(Fork 6R Position) -> Fork 6R Position [‰]/1
  Gear Sets/3(Fork N5 Position) -> Fork N5 Position [‰]/1
  Data Type Conversion/1 -> Product/2
  Engine/1(Engine Throttle [%]) -> Engine Throttle [%]/1
  Engine/4(Engine Consumption Rate [g/s]) -> Engine Consumption Rate [g/s]/1
  connections:
  Dual Clutch/LConn1 -- Engine/RConn1
  Gear Sets/LConn1 -- Ideal Rotational Motion Sensor/LConn1 -- Dual Clutch/RConn1
  Gear Sets/LConn2 -- Dual Clutch/RConn2 -- Ideal Rotational Motion Sensor1/LConn1
  Ideal Torque Sensor/LConn1 -- Gear Sets/RConn1
  Ideal Rotational Motion Sensor/RConn1 -- Mechanical Rotational Reference/LConn1
  Ideal Rotational Motion Sensor/RConn2 -- PS-Simulink Converter/LConn1
  Ideal Rotational Motion Sensor1/RConn1 -- Mechanical Rotational Reference1/LConn1
  Ideal Rotational Motion Sensor1/RConn2 -- PS-Simulink Converter1/LConn1
  Ideal Torque Sensor/RConn2 -- PS-Simulink Converter3/LConn1
  Ideal Torque Sensor/RConn1 -- Output Shaft/RConn1

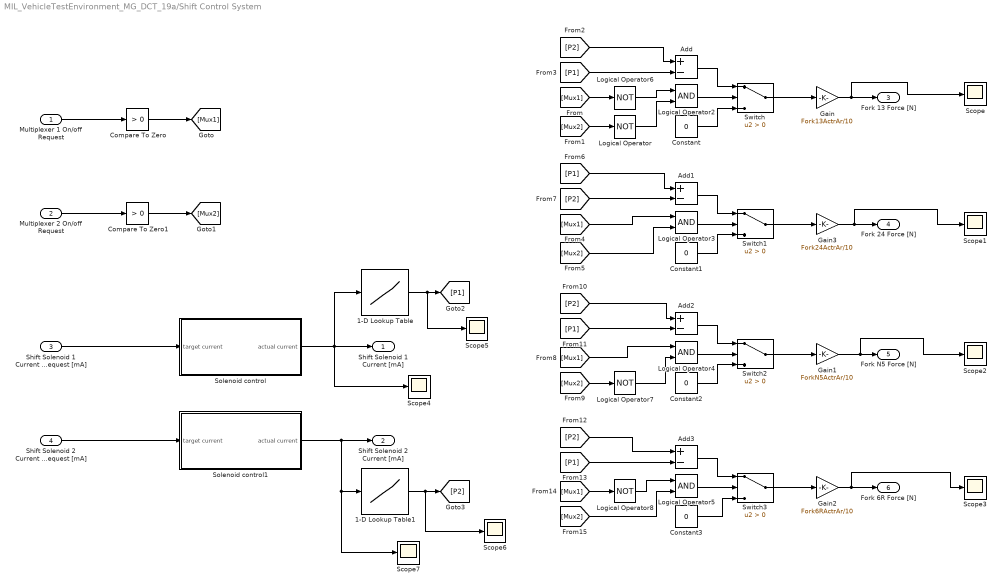
== system MIL_VehicleTestEnvironment_MG_DCT_19a/Shift Control System ==
  Multiplexer 1 On/off Request : Inport
  Multiplexer 2 On/off Request : Inport  Port=2
  Shift Solenoid 1 Current Request [mA] : Inport  Port=3
  Shift Solenoid 2 Current Request [mA] : Inport  Port=4
  1-D Lookup Table : Lookup_n-D  NumberOfTableDimensions=1  BreakpointsForDimension1=ShiftSoln1LineI  Table=ShiftSoln1LineP  ExtrapMethod=Clip  InternalRulePriority=Speed  RndMeth=Simplest  InputSameDT=on
  1-D Lookup Table1 : Lookup_n-D  NumberOfTableDimensions=1  BreakpointsForDimension1=ShiftSoln2LineI  Table=ShiftSoln2LineP  ExtrapMethod=Clip  InternalRulePriority=Speed  RndMeth=Simplest  InputSameDT=on
  Add{,1..3} (4 alike) : Sum  Inputs=+-
  Compare To Zero : simulink/Logic and Bit Operations/Compare To Zero  relop=>  OutDataTypeStr=boolean
  Compare To Zero1 : simulink/Logic and Bit Operations/Compare To Zero  relop=>  OutDataTypeStr=boolean
  Constant{,1..3} (4 alike) : Constant  Value=0
  Gain : Gain  Gain=Fork13ActrAr/10
  Gain1 : Gain  Gain=ForkN5ActrAr/10
  Gain2 : Gain  Gain=Fork6RActrAr/10
  Gain3 : Gain  Gain=Fork24ActrAr/10
  Logical Operator{,6..8} (4 alike) : Logic  Operator=NOT  AllPortsSameDT=off  OutDataTypeStr=boolean
  Logical Operator{2..5} (4 alike) : Logic  AllPortsSameDT=off  OutDataTypeStr=boolean
  Scope{,1..7} (8 alike) : Scope
  Solenoid control : Subsystem
  Solenoid control1 : Subsystem
  Switch{,1..3} (4 alike) : Switch  Criteria=u2 > Threshold
  Shift Solenoid 1 Current [mA] : Outport  VectorParamsAs1DForOutWhenUnconnected=off
  Shift Solenoid 2 Current [mA] : Outport  Port=2  VectorParamsAs1DForOutWhenUnconnected=off
  Fork 13 Force [N] : Outport  Port=3  VectorParamsAs1DForOutWhenUnconnected=off
  Fork 24 Force [N] : Outport  Port=4  VectorParamsAs1DForOutWhenUnconnected=off
  Fork N5 Force [N] : Outport  Port=5  VectorParamsAs1DForOutWhenUnconnected=off
  Fork 6R Force [N] : Outport  Port=6  VectorParamsAs1DForOutWhenUnconnected=off
  wires:
  Shift Solenoid 1 Current Request [mA]/1 -> Solenoid control/1(target current)
  Shift Solenoid 2 Current Request [mA]/1 -> Solenoid control1/1(target current)
  Solenoid control/1(actual current) -> Scope4/1, Shift Solenoid 1 Current [mA]/1, 1-D Lookup Table/1
  Solenoid control1/1(actual current) -> Shift Solenoid 2 Current [mA]/1, Scope7/1, 1-D Lookup Table1/1
  Gain1/1 -> Scope2/1, Fork N5 Force [N]/1
  Gain/1 -> Scope/1, Fork 13 Force [N]/1
  Gain2/1 -> Scope3/1, Fork 6R Force [N]/1
  Gain3/1 -> Scope1/1, Fork 24 Force [N]/1
  Multiplexer 1 On/off Request/1 -> Compare To Zero/1
  Multiplexer 2 On/off Request/1 -> Compare To Zero1/1
  Logical Operator2/1 -> Switch/2
  Switch/1 -> Gain/1
  Logical Operator3/1 -> Switch1/2
  Switch1/1 -> Gain3/1
  Logical Operator4/1 -> Switch2/2
  Switch2/1 -> Gain1/1
  Logical Operator5/1 -> Switch3/2
  Switch3/1 -> Gain2/1
  Compare To Zero/1 -> [Mux1]
  Compare To Zero1/1 -> [Mux2]
  1-D Lookup Table/1 -> Scope5/1, [P1]
  1-D Lookup Table1/1 -> Scope6/1, [P2]
  [Mux2] -> Logical Operator/1
  [Mux1] -> Logical Operator6/1
  Logical Operator6/1 -> Logical Operator2/1
  Logical Operator/1 -> Logical Operator2/2
  [P2] -> Add/1
  [P1] -> Add/2
  [P1] -> Add1/1
  [P2] -> Add1/2
  [Mux1] -> Logical Operator3/1
  [Mux2] -> Logical Operator3/2
  [P2] -> Add2/1
  [P1] -> Add2/2
  [Mux2] -> Logical Operator7/1
  [Mux1] -> Logical Operator4/1
  [P2] -> Add3/1
  [P1] -> Add3/2
  Logical Operator8/1 -> Logical Operator5/1
  [Mux2] -> Logical Operator5/2
  Add/1 -> Switch/1
  Constant/1 -> Switch/3
  Constant1/1 -> Switch1/3
  Add1/1 -> Switch1/1
  Add2/1 -> Switch2/1
  Constant2/1 -> Switch2/3
  Constant3/1 -> Switch3/3
  Add3/1 -> Switch3/1
  Logical Operator7/1 -> Logical Operator4/2
  [Mux1] -> Logical Operator8/1

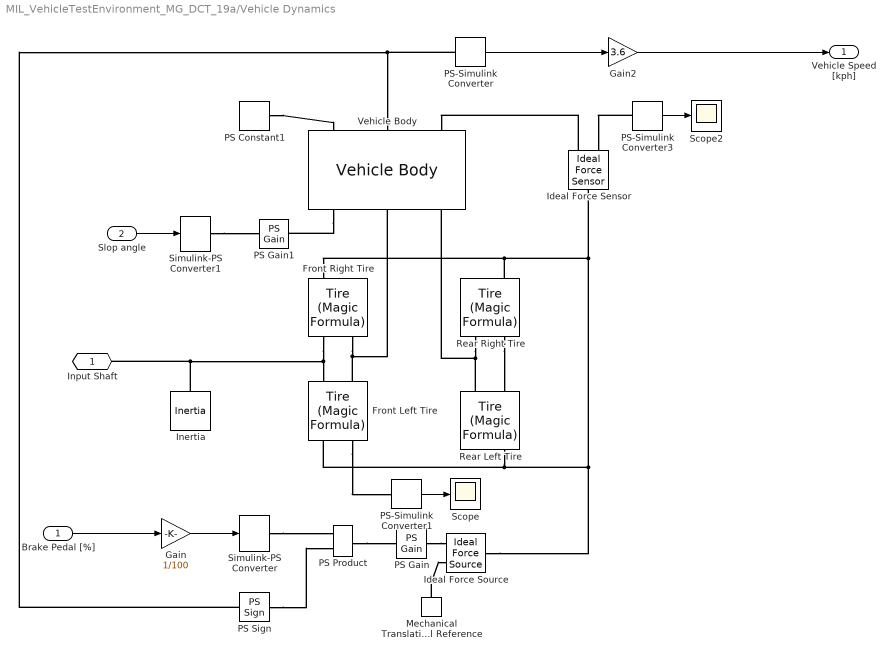
== system MIL_VehicleTestEnvironment_MG_DCT_19a/Vehicle Dynamics ==
  Brake Pedal [%] : Inport
  Slop angle : Inport  Port=2
  Front Left Tire : sdl_lib/Tires & Vehicles/Tire (Magic Formula)  parameterization=3  F_z1=TireLoadRatd N  F_x1=TireForMax N  kappa1=TireSlipPeak  B_m=10  C_m=1.9  D_m=1  E_m=0.97  fz0=4e+3 N  p_Cx=1.685  p_Dx=[ 5 -0.037 ]  p_Ex=[ 0.344 0.095 -0.02 0 ]  p_Kx=[ 21.51 -0.163 0.245 ]  p_Hx=[ -0.002 0.002 ]  p_Vx=[ 0 0 ]  v_tr_thr=0.1 m/s  r_e=TireRad m  model_compliance=0  stiffness=1e+6 N/m  damping=1000 N/(m/s)  model_inertia=1  inertia=WhlInrt kg*m^2  initial_velocity=0 rad/s  model_resistance=1  resistance_model=1  coeff=TireRollRest  p_tire=250e3 Pa  alpha=-0.003  beta=0.97  coeff_a=84e-4  coeff_b=6.2e-4 s/m  coeff_c=1.6e-4 s^2/m^2  v_thr=1e-3 m/s
  Front Right Tire : sdl_lib/Tires & Vehicles/Tire (Magic Formula)  parameterization=3  F_z1=TireLoadRatd N  F_x1=TireForMax N  kappa1=TireSlipPeak  B_m=10  C_m=1.9  D_m=1  E_m=0.97  fz0=4e+3 N  p_Cx=1.685  p_Dx=[ 5 -0.037 ]  p_Ex=[ 0.344 0.095 -0.02 0 ]  p_Kx=[ 21.51 -0.163 0.245 ]  p_Hx=[ -0.002 0.002 ]  p_Vx=[ 0 0 ]  v_tr_thr=0.1 m/s  r_e=TireRad m  model_compliance=0  stiffness=1e+6 N/m  damping=1000 N/(m/s)  model_inertia=1  inertia=WhlInrt kg*m^2  initial_velocity=0 rad/s  model_resistance=1  resistance_model=1  coeff=TireRollRest  p_tire=250e3 Pa  alpha=-0.003  beta=0.97  coeff_a=84e-4  coeff_b=6.2e-4 s/m  coeff_c=1.6e-4 s^2/m^2  v_thr=1e-3 m/s
  Gain : Gain  Gain=1/100
  Gain2 : Gain  Gain=3.6
  Ideal Force Sensor : fl_lib/Mechanical/Mechanical Sensors/Ideal Force Sensor
  Ideal Force Source : fl_lib/Mechanical/Mechanical Sources/Ideal Force Source
  Inertia : fl_lib/Mechanical/Rotational Elements/Inertia  inertia=HalfShafInrt*2 kg*m^2  w_specify=off  w_priority=High  w=0 rad/s  w_nominal_specify=off  w_nominal_unit=rad/s  w_nominal_value=1  t_specify=off  t_priority=High  t=0 N*m  t_nominal_specify=off  t_nominal_unit=N*m  t_nominal_value=1
  Mechanical Translational Reference : fl_lib/Mechanical/Translational Elements/Mechanical Translational Reference
  PS Constant1 : fl_lib/Physical Signals/Sources/PS Constant  constant=0
  PS Gain : fl_ps_legacy_lib/Legacy Physical Signals/Functions/PS Gain  gain=-VehDecMax*VehMass
  PS Gain1 : fl_ps_legacy_lib/Legacy Physical Signals/Functions/PS Gain  gain=1
  PS Product : fl_ps_legacy_lib/Legacy Physical Signals/Functions/PS Product
      settings: SourceProductBaseCode=SS
  PS Sign : fl_ps_legacy_lib/Legacy Physical Signals/Nonlinear Operators/PS Sign
      settings: SourceProductBaseCode=SS  InternalSimscapePortConfiguration="{\"Bottom\":[],\"Left\":[{\"id\":\"I\",\"label\":\"\",\"type\":\"input\"}],\"Right\":[{\"id\":\"O\",\"label\":\"\",\"type\":\"output\"}],\"Top\":[]}"
  PS-Simulink Converter : nesl_utility/PS-Simulink Converter  PhysicalDomain=network_engine_domain  SubClassName=ps_output  LeftPortType=input  RightPortType=output  PseudoPeriodic=off  Frequencies=[]  Unit=m/s  AffineConversion=off
  PS-Simulink Converter1 : nesl_utility/PS-Simulink Converter  PhysicalDomain=network_engine_domain  SubClassName=ps_output  LeftPortType=input  RightPortType=output  PseudoPeriodic=off  Frequencies=[]  Unit=1  AffineConversion=off
  PS-Simulink Converter3 : nesl_utility/PS-Simulink Converter  PhysicalDomain=network_engine_domain  SubClassName=ps_output  LeftPortType=input  RightPortType=output  PseudoPeriodic=off  Frequencies=[]  Unit=N  AffineConversion=off
  Rear Left Tire : sdl_lib/Tires & Vehicles/Tire (Magic Formula)  parameterization=3  F_z1=TireLoadRatd N  F_x1=TireForMax N  kappa1=TireSlipPeak  B_m=10  C_m=1.9  D_m=1  E_m=0.97  fz0=4e+3 N  p_Cx=1.685  p_Dx=[ 1.21 -0.037 ]  p_Ex=[ 0.344 0.095 -0.02 0 ]  p_Kx=[ 21.51 -0.163 0.245 ]  p_Hx=[ -0.002 0.002 ]  p_Vx=[ 0 0 ]  v_tr_thr=0.1 m/s  r_e=TireRad m  model_compliance=0  stiffness=1e+6 N/m  damping=1000 N/(m/s)  model_inertia=1  inertia=WhlInrt kg*m^2  initial_velocity=0 rad/s  model_resistance=1  resistance_model=1  coeff=TireRollRest  p_tire=250e3 Pa  alpha=-0.003  beta=0.97  coeff_a=84e-4  coeff_b=6.2e-4 s/m  coeff_c=1.6e-4 s^2/m^2  v_thr=1e-3 m/s
  Rear Right Tire : sdl_lib/Tires & Vehicles/Tire (Magic Formula)  parameterization=3  F_z1=TireLoadRatd N  F_x1=TireForMax N  kappa1=TireSlipPeak  B_m=10  C_m=1.9  D_m=1  E_m=0.97  fz0=4e+3 N  p_Cx=1.685  p_Dx=[ 1.21 -0.037 ]  p_Ex=[ 0.344 0.095 -0.02 0 ]  p_Kx=[ 21.51 -0.163 0.245 ]  p_Hx=[ -0.002 0.002 ]  p_Vx=[ 0 0 ]  v_tr_thr=0.1 m/s  r_e=TireRad m  model_compliance=0  stiffness=1e+6 N/m  damping=1000 N/(m/s)  model_inertia=1  inertia=WhlInrt kg*m^2  initial_velocity=0 rad/s  model_resistance=1  resistance_model=1  coeff=TireRollRest  p_tire=250e3 Pa  alpha=-0.003  beta=0.97  coeff_a=84e-4  coeff_b=6.2e-4 s/m  coeff_c=1.6e-4 s^2/m^2  v_thr=1e-3 m/s
  Scope : Scope
  Scope2 : Scope
  Simulink-PS Converter : nesl_utility/Simulink-PS Converter  PhysicalDomain=network_engine_domain  SubClassName=ps_input  LeftPortType=input  RightPortType=output  PseudoPeriodic=off  Frequencies=[]  NoiseDistribution=none  NoiseParameters=[]  Unit=1  AffineConversion=off  FilteringAndDerivatives=zero  SimscapeFilterOrder=1  InputFilterTimeConstant=0.001  UdotUserProvided=1
  Simulink-PS Converter1 : nesl_utility/Simulink-PS Converter  PhysicalDomain=network_engine_domain  SubClassName=ps_input  LeftPortType=input  RightPortType=output  PseudoPeriodic=off  Frequencies=[]  NoiseDistribution=none  NoiseParameters=[]  Unit=deg  AffineConversion=off  FilteringAndDerivatives=zero  SimscapeFilterOrder=1  InputFilterTimeConstant=0.001  UdotUserProvided=1
  Vehicle Body : sdl_lib/Tires & Vehicles/Vehicle Body  mass=VehMass kg  n_w=2  x_f=CGFrntAxleDist m  x_r=CGRearAxleDist m  y_c=CGHght m  mass_var=simscape.enum.onoff.off  model_pitch=simscape.enum.onoff.off  inertia=4000 kg*m^2  suspension_model=sdl.enum.linearTLU.linear  k_f=1e4 N/m  b_f=1e4 N/(m/s)  k_r=1e4 N/m  b_r=1e4 N/(m/s)  k_f_TLU=[-2000, -1000, 0, 1000, 2000] N  x_f_TLU=[-.4, -.2, 0, .2, .4] m  b_f_TLU=[-200, -100, 0, 100, 200] N  v_f_TLU=[-4, -2, 0, 2, 4] m/s  k_r_TLU=[-2000, -1000, 0, 1000, 2000] N  x_r_TLU=[-.4, -.2, 0, .2, .4] m  b_r_TLU=[-200, -100, 0, 100, 200] N  v_r_TLU=[-4, -2, 0, 2, 4] m/s  interp_method=simscape.enum.interpolation.linear  extrap_method=simscape.enum.extrapolation.linear  model_hardstop=simscape.enum.onoff.off  upper_bound_f=.25 m  lower_bound_f=-.25 m  stop_k_f=1e6 N/m  stop_b_f=150 N/(m/s)  upper_bound_r=.25 m  lower_bound_r=-.25 m  stop_k_r=1e6 N/m  stop_b_r=150 N/(m/s)  initial_pitch=0 rad  initial_pitch_rate=0 rad/s  g=9.81 m/s^2  liftoff_warning=simscape.enum.onoff.off  area=VehFrntArea m^2  Cd=VehAirDragCoef  rho=1.18 kg/m^3  v_specify=on  v_priority=High  v=VehSpdInit m/s  v_nominal_specify=off  v_nominal_unit=m/s  v_nominal_value=1
  Input Shaft : PMIOPort  Side=Left
  Vehicle Speed [kph] : Outport  VectorParamsAs1DForOutWhenUnconnected=off
  wires:
  PS-Simulink Converter/1 -> Gain2/1
  Gain2/1 -> Vehicle Speed [kph]/1
  Brake Pedal [%]/1 -> Gain/1
  Gain/1 -> Simulink-PS Converter/1
  Slop angle/1 -> Simulink-PS Converter1/1
  PS-Simulink Converter1/1 -> Scope/1
  PS-Simulink Converter3/1 -> Scope2/1
  connections:
  Rear Right Tire/LConn2 -- Rear Left Tire/LConn2
  Vehicle Body/RConn3 -- PS Gain1/RConn1
  PS Constant1/RConn1 -- Vehicle Body/LConn3
  Mechanical Translational Reference/LConn1 -- Ideal Force Source/RConn2
  PS-Simulink Converter/LConn1 -- PS Sign/LConn1 -- Vehicle Body/LConn2
  PS Gain/RConn1 -- Ideal Force Source/RConn1
  Simulink-PS Converter/RConn1 -- PS Product/LConn1
  PS Sign/RConn1 -- PS Product/LConn2
  PS Product/RConn1 -- PS Gain/LConn1
  Simulink-PS Converter1/RConn1 -- PS Gain1/LConn1
  Front Left Tire/RConn1 -- PS-Simulink Converter1/LConn1
  Inertia/LConn1 -- Front Left Tire/LConn2 -- Front Right Tire/LConn2 -- Input Shaft/RConn1
  Rear Left Tire/LConn1 -- Rear Right Tire/LConn1 -- Vehicle Body/RConn1
  Front Left Tire/LConn1 -- Vehicle Body/RConn2 -- Front Right Tire/LConn1
  PS-Simulink Converter3/LConn1 -- Ideal Force Sensor/RConn2
  Ideal Force Sensor/RConn1 -- Vehicle Body/LConn1
  Ideal Force Source/LConn1 -- Rear Left Tire/RConn2 -- Front Left Tire/RConn2 -- Rear Right Tire/RConn2 -- Front Right Tire/RConn2 -- Ideal Force Sensor/LConn1

== system MIL_VehicleTestEnvironment_MG_DCT_19a/Clutch Control System/Solenoid control ==
  target current : Inport
  Constant : Constant  Value=13/VFS1R*1000
  MinMax : MinMax  Inputs=2
  actual current : Outport  VectorParamsAs1DForOutWhenUnconnected=off
  wires:
  Constant/1 -> MinMax/2
  target current/1 -> MinMax/1
  MinMax/1 -> actual current/1

== system MIL_VehicleTestEnvironment_MG_DCT_19a/Clutch Control System/Solenoid control1 ==
  target current : Inport
  Constant : Constant  Value=13/VFS2R*1000
  MinMax : MinMax  Inputs=2
  actual current : Outport  VectorParamsAs1DForOutWhenUnconnected=off
  wires:
  Constant/1 -> MinMax/2
  target current/1 -> MinMax/1
  MinMax/1 -> actual current/1

== system MIL_VehicleTestEnvironment_MG_DCT_19a/Main Line & Lube Control System/Solenoid control ==
  target current : Inport
  Constant : Constant  Value=13/VBS3R*1000
  MinMax : MinMax  Inputs=2
  actual current : Outport  VectorParamsAs1DForOutWhenUnconnected=off
  wires:
  Constant/1 -> MinMax/2
  target current/1 -> MinMax/1
  MinMax/1 -> actual current/1

== system MIL_VehicleTestEnvironment_MG_DCT_19a/Main Line & Lube Control System/Solenoid control1 ==
  target current : Inport
  Constant : Constant  Value=13/VBS4R*1000
  MinMax : MinMax  Inputs=2
  actual current : Outport  VectorParamsAs1DForOutWhenUnconnected=off
  wires:
  Constant/1 -> MinMax/2
  target current/1 -> MinMax/1
  MinMax/1 -> actual current/1

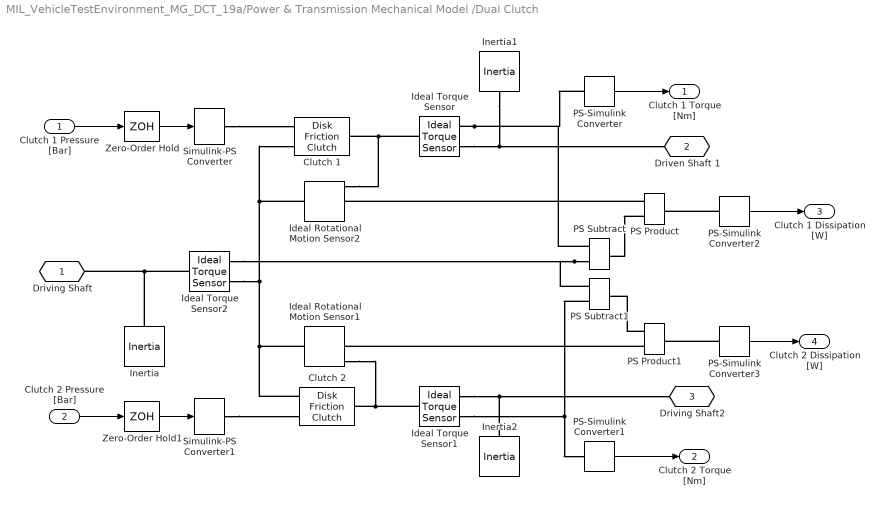
== system MIL_VehicleTestEnvironment_MG_DCT_19a/Power & Transmission Mechanical Model /Dual Clutch ==
  Clutch 1 Pressure [Bar] : Inport
  Clutch 2 Pressure [Bar] : Inport  Port=2
  Clutch 1 : sdl_lib/Clutches/Disk Friction Clutch  geometry_model=1  r_eff=Clu1EffRad m  d_o=150 mm  d_i=100 mm  nS=Clu1FricSurfNum  piston_area=Clu1PresArea m^2  unidirectional=0  friction_model=2  mu_w_vector=Clu1FricCoefMap(:,1) rpm  temperature_TLU=[280, 300, 320] K  mu_static=Clu1StatFricCoef  mu_static_vector=[.4, .38, .36]  mu_coulomb=Clu1StatFricCoef  mu_coulomb_vector=Clu1FricCoefMap(:,2)  mu_coulomb_temp_vector=[.3, .28, .25]  mu_coulomb_matrix=[.34, .32, .3; .3, .28, .25; .25, .2, .15]  mu_interp_method=1  mu_extrap_method=1  d_f=1  w_tol=0.001 rad/s  pressure_min=Clu1PMin bar  mu_visc=0 N*m/(rad/s)  initial_state_locked=0  thermal_mass=25 kJ/K  T_init=300 K
      settings: SourceProductBaseCode=LD  InternalSimscapePortConfiguration="{\"Bottom\":[],\"Left\":[{\"id\":\"P\",\"label\":\"P\",\"type\":\"input\"},{\"id\":\"B\",\"label\":\"B\",\"type\":\"foundation.mechanical.rotational.rotational\"}],\"Right\":[{\"id\":\"F\",\"label\":\"F\",\"type\":\"foundation.mechanical.rotational.rotational\"}],\"Top\":[]}"
  Clutch 2 : sdl_lib/Clutches/Disk Friction Clutch  geometry_model=1  r_eff=Clu2EffRad m  d_o=150 mm  d_i=100 mm  nS=Clu2FricSurfNum  piston_area=Clu2PresArea m^2  unidirectional=0  friction_model=2  mu_w_vector=Clu2FricCoefMap(:,1) rpm  temperature_TLU=[280, 300, 320] K  mu_static=Clu2StatFricCoef  mu_static_vector=[.4, .38, .36]  mu_coulomb=Clu2StatFricCoef  mu_coulomb_vector=Clu2FricCoefMap(:,2)  mu_coulomb_temp_vector=[.3, .28, .25]  mu_coulomb_matrix=[.34, .32, .3; .3, .28, .25; .25, .2, .15]  mu_interp_method=1  mu_extrap_method=1  d_f=1  w_tol=0.001 rad/s  pressure_min=Clu2PMin bar  mu_visc=0 N*m/(rad/s)  initial_state_locked=0  thermal_mass=25 kJ/K  T_init=300 K
      settings: SourceProductBaseCode=LD  InternalSimscapePortConfiguration="{\"Bottom\":[],\"Left\":[{\"id\":\"P\",\"label\":\"P\",\"type\":\"input\"},{\"id\":\"B\",\"label\":\"B\",\"type\":\"foundation.mechanical.rotational.rotational\"}],\"Right\":[{\"id\":\"F\",\"label\":\"F\",\"type\":\"foundation.mechanical.rotational.rotational\"}],\"Top\":[]}"
  Ideal Rotational Motion Sensor1 : fl_lib/Mechanical/Mechanical Sensors/Ideal Rotational Motion Sensor  wrap_angle=simscape.enum.onoff.off  offset=0 rad
  Ideal Rotational Motion Sensor2 : fl_lib/Mechanical/Mechanical Sensors/Ideal Rotational Motion Sensor  wrap_angle=simscape.enum.onoff.off  offset=0 rad
  Ideal Torque Sensor : fl_lib/Mechanical/Mechanical Sensors/Ideal Torque Sensor
  Ideal Torque Sensor1 : fl_lib/Mechanical/Mechanical Sensors/Ideal Torque Sensor
  Ideal Torque Sensor2 : fl_lib/Mechanical/Mechanical Sensors/Ideal Torque Sensor
  Inertia : fl_lib/Mechanical/Rotational Elements/Inertia  inertia=CluInpInrt kg*m^2  w_specify=off  w_priority=High  w=0 rad/s  w_nominal_specify=off  w_nominal_unit=rad/s  w_nominal_value=1  t_specify=off  t_priority=High  t=0 N*m  t_nominal_specify=off  t_nominal_unit=N*m  t_nominal_value=1
  Inertia1 : fl_lib/Mechanical/Rotational Elements/Inertia  inertia=Clu1OutpInrt kg*m^2  w_specify=off  w_priority=High  w=0 rad/s  w_nominal_specify=off  w_nominal_unit=rad/s  w_nominal_value=1  t_specify=off  t_priority=High  t=0 N*m  t_nominal_specify=off  t_nominal_unit=N*m  t_nominal_value=1
  Inertia2 : fl_lib/Mechanical/Rotational Elements/Inertia  inertia=Clu2OutpInrt kg*m^2  w_specify=off  w_priority=High  w=0 rad/s  w_nominal_specify=off  w_nominal_unit=rad/s  w_nominal_value=1  t_specify=off  t_priority=High  t=0 N*m  t_nominal_specify=off  t_nominal_unit=N*m  t_nominal_value=1
  PS Product : fl_ps_legacy_lib/Legacy Physical Signals/Functions/PS Product
      settings: SourceProductBaseCode=SS
  PS Product1 : fl_ps_legacy_lib/Legacy Physical Signals/Functions/PS Product
      settings: SourceProductBaseCode=SS
  PS Subtract : fl_ps_legacy_lib/Legacy Physical Signals/Functions/PS Subtract
      settings: SourceProductBaseCode=SS
  PS Subtract1 : fl_ps_legacy_lib/Legacy Physical Signals/Functions/PS Subtract
      settings: SourceProductBaseCode=SS
  PS-Simulink Converter : nesl_utility/PS-Simulink Converter  PhysicalDomain=network_engine_domain  SubClassName=ps_output  LeftPortType=input  RightPortType=output  PseudoPeriodic=off  Frequencies=[]  Unit=N*m  AffineConversion=off
  PS-Simulink Converter1 : nesl_utility/PS-Simulink Converter  PhysicalDomain=network_engine_domain  SubClassName=ps_output  LeftPortType=input  RightPortType=output  PseudoPeriodic=off  Frequencies=[]  Unit=N*m  AffineConversion=off
  PS-Simulink Converter2 : nesl_utility/PS-Simulink Converter  PhysicalDomain=network_engine_domain  SubClassName=ps_output  LeftPortType=input  RightPortType=output  PseudoPeriodic=off  Frequencies=[]  Unit=J/s  AffineConversion=off
  PS-Simulink Converter3 : nesl_utility/PS-Simulink Converter  PhysicalDomain=network_engine_domain  SubClassName=ps_output  LeftPortType=input  RightPortType=output  PseudoPeriodic=off  Frequencies=[]  Unit=J/s  AffineConversion=off
  Simulink-PS Converter : nesl_utility/Simulink-PS Converter  PhysicalDomain=network_engine_domain  SubClassName=ps_input  LeftPortType=input  RightPortType=output  PseudoPeriodic=off  Frequencies=[]  NoiseDistribution=none  NoiseParameters=[]  Unit=bar  AffineConversion=off  FilteringAndDerivatives=zero  SimscapeFilterOrder=1  InputFilterTimeConstant=0.001  UdotUserProvided=1
  Simulink-PS Converter1 : nesl_utility/Simulink-PS Converter  PhysicalDomain=network_engine_domain  SubClassName=ps_input  LeftPortType=input  RightPortType=output  PseudoPeriodic=off  Frequencies=[]  NoiseDistribution=none  NoiseParameters=[]  Unit=bar  AffineConversion=off  FilteringAndDerivatives=zero  SimscapeFilterOrder=1  InputFilterTimeConstant=0.001  UdotUserProvided=1
  Zero-Order Hold : ZeroOrderHold  SampleTime=0.001
  Zero-Order Hold1 : ZeroOrderHold  SampleTime=0.001
  Driving Shaft : PMIOPort  Side=Left
  Driven Shaft 1 : PMIOPort  Port=2  Side=Right
  Driving Shaft2 : PMIOPort  Port=3  Side=Right
  Clutch 1 Torque [Nm] : Outport  VectorParamsAs1DForOutWhenUnconnected=off
  Clutch 2 Torque [Nm] : Outport  Port=2  VectorParamsAs1DForOutWhenUnconnected=off
  Clutch 1 Dissipation [W] : Outport  Port=3  VectorParamsAs1DForOutWhenUnconnected=off
  Clutch 2 Dissipation [W] : Outport  Port=4  VectorParamsAs1DForOutWhenUnconnected=off
  wires:
  Clutch 1 Pressure [Bar]/1 -> Zero-Order Hold/1
  Clutch 2 Pressure [Bar]/1 -> Zero-Order Hold1/1
  PS-Simulink Converter/1 -> Clutch 1 Torque [Nm]/1
  PS-Simulink Converter1/1 -> Clutch 2 Torque [Nm]/1
  PS-Simulink Converter2/1 -> Clutch 1 Dissipation [W]/1
  PS-Simulink Converter3/1 -> Clutch 2 Dissipation [W]/1
  Zero-Order Hold/1 -> Simulink-PS Converter/1
  Zero-Order Hold1/1 -> Simulink-PS Converter1/1
  connections:
  Simulink-PS Converter/RConn1 -- Clutch 1/LConn1
  Ideal Rotational Motion Sensor1/LConn1 -- Clutch 2/LConn2 -- Ideal Torque Sensor2/RConn1 -- Ideal Rotational Motion Sensor2/LConn1 -- Clutch 1/LConn2
  Simulink-PS Converter1/RConn1 -- Clutch 2/LConn1
  Ideal Torque Sensor/LConn1 -- Ideal Rotational Motion Sensor2/RConn1 -- Clutch 1/RConn1
  Ideal Torque Sensor1/LConn1 -- Ideal Rotational Motion Sensor1/RConn1 -- Clutch 2/RConn1
  Ideal Torque Sensor/RConn2 -- PS-Simulink Converter/LConn1 -- PS Subtract/LConn2
  PS Subtract1/LConn2 -- Ideal Torque Sensor1/RConn2 -- PS-Simulink Converter1/LConn1
  Ideal Torque Sensor1/RConn1 -- Inertia2/LConn1 -- Driving Shaft2/RConn1
  Ideal Torque Sensor/RConn1 -- Inertia1/LConn1 -- Driven Shaft 1/RConn1
  Ideal Torque Sensor2/LConn1 -- Inertia/LConn1 -- Driving Shaft/RConn1
  PS Subtract/LConn1 -- Ideal Torque Sensor2/RConn2 -- PS Subtract1/LConn1
  PS Product/LConn1 -- Ideal Rotational Motion Sensor2/RConn2
  PS Product/LConn2 -- PS Subtract/RConn1
  PS-Simulink Converter2/LConn1 -- PS Product/RConn1
  PS Product1/LConn1 -- PS Subtract1/RConn1
  PS Product1/LConn2 -- Ideal Rotational Motion Sensor1/RConn2
  PS-Simulink Converter3/LConn1 -- PS Product1/RConn1

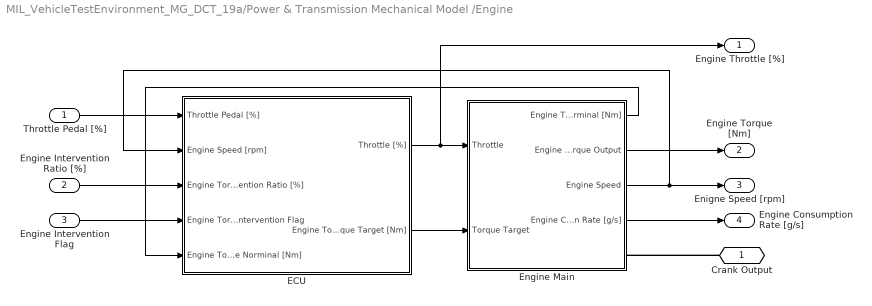
== system MIL_VehicleTestEnvironment_MG_DCT_19a/Power & Transmission Mechanical Model /Engine ==
  Throttle Pedal [%] : Inport
  Engine Intervention Ratio [%] : Inport  Port=2
  Engine Intervention Flag : Inport  Port=3
  ECU : Subsystem
  Engine Main : Subsystem
  Crank Output : PMIOPort  Side=Right
  Engine Throttle [%] : Outport  VectorParamsAs1DForOutWhenUnconnected=off
  Engine Torque [Nm] : Outport  Port=2  VectorParamsAs1DForOutWhenUnconnected=off
  Enigne Speed [rpm] : Outport  Port=3  VectorParamsAs1DForOutWhenUnconnected=off
  Engine Consumption Rate [g/s] : Outport  Port=4  VectorParamsAs1DForOutWhenUnconnected=off
  wires:
  Engine Main/2(Engine Torque Output) -> Engine Torque [Nm]/1
  Engine Intervention Flag/1 -> ECU/4(Engine Torque Intervention Flag)
  Engine Intervention Ratio [%]/1 -> ECU/3(Engine Torque Intervention Ratio [%])
  Throttle Pedal [%]/1 -> ECU/1(Throttle Pedal [%])
  ECU/1(Throttle [%]) -> Engine Throttle [%]/1, Engine Main/1(Throttle)
  ECU/2("Engine Torque Target [Nm] ") -> Engine Main/2(Torque Target)
  Engine Main/3(Engine Speed) -> Enigne Speed [rpm]/1, ECU/2(Engine Speed [rpm])
  Engine Main/1(Engine Torque Norminal [Nm]) -> ECU/5(Engine Torque Norminal [Nm])
  Engine Main/4(Engine Consumption Rate [g/s]) -> Engine Consumption Rate [g/s]/1
  connections:
  Crank Output/RConn1 -- Engine Main/RConn1
